simulink model "smc"  (R2015b)
settings: Solver=ode4  StartTime=0.0  StopTime=20  FixedStep=0.0001  RelTol=1e-3
values from neighbouring files (symbols this model uses):
  L = 1    [init.m]
  r = 1    [init.m]
libraries: simulink x1
settings Model: Creator=Subodh  LastModifiedBy=Subodh
settings HardwareCC: ProdWordSize=32  ProdHWDeviceType=Specified

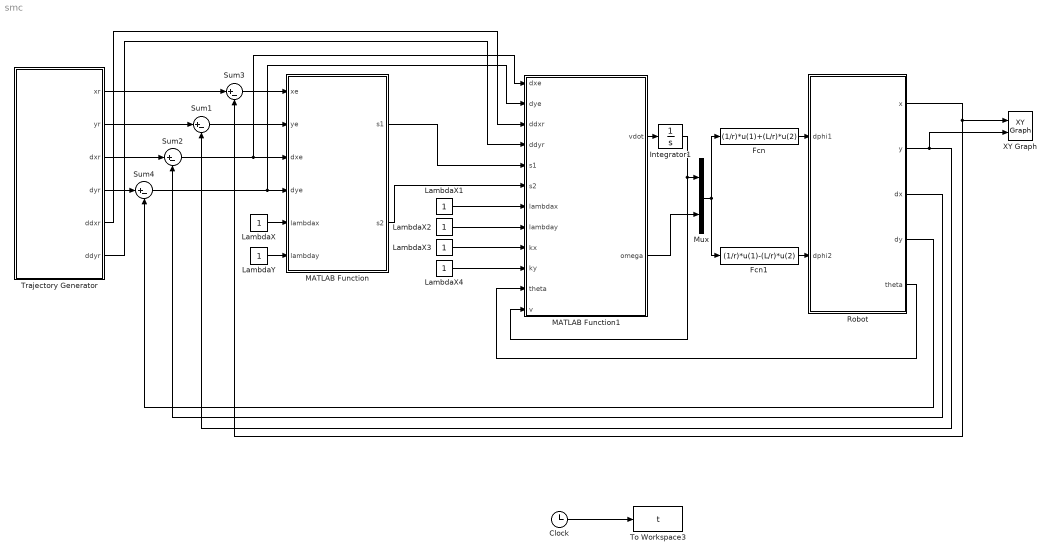
== system smc ==
  "                               LambdaX1" : Constant
  "                               LambdaX2" : Constant
  "                             LambdaX3" : Constant
  "                            LambdaX4" : Constant
  Clock : Clock
  Fcn : Fcn  Expr=(1/r)*u(1)+(L/r)*u(2)
  Fcn1 : Fcn  Expr=(1/r)*u(1)-(L/r)*u(2)
  Integrator1 : Integrator  InitialCondition=1
  LambdaX : Constant
  LambdaY : Constant
  MATLAB Function : MATLAB Function  TreatAsAtomicUnit=on
  MATLAB Function1 : MATLAB Function  TreatAsAtomicUnit=on
  Mux : Mux  Inputs=2
  Robot : Subsystem
  Sum{1..4} (4 alike) : Sum  Inputs=|+-
  To Workspace3 : ToWorkspace  VariableName=t  SampleTime=-1
  Trajectory Generator : Subsystem
  XY Graph : simulink/Sinks/XY Graph  xmin=-2  xmax=2  ymin=-2  ymax=2  st=-1
  wires:
  Clock/1 -> To Workspace3/1
  Trajectory Generator/1(xr) -> Sum3/1
  Robot/1(x) -> XY Graph/1, Sum3/2
  Trajectory Generator/2(yr) -> Sum1/1
  Robot/2(y) -> XY Graph/2, Sum1/2
  Trajectory Generator/3(dxr) -> Sum2/1
  Robot/3(dx) -> Sum2/2
  Trajectory Generator/4(dyr) -> Sum4/1
  Robot/4(dy) -> Sum4/2
  Sum1/1 -> MATLAB Function/2(ye)
  Sum3/1 -> MATLAB Function/1(xe)
  Sum2/1 -> MATLAB Function1/1(dxe), MATLAB Function/3(dxe)
  Sum4/1 -> MATLAB Function1/2(dye), MATLAB Function/4(dye)
  LambdaX/1 -> MATLAB Function/5(lambdax)
  LambdaY/1 -> MATLAB Function/6(lambday)
  MATLAB Function1/1(vdot) -> Integrator1/1
  Integrator1/1 -> Mux/1, MATLAB Function1/12(v)
  Trajectory Generator/5(ddxr) -> MATLAB Function1/3(ddxr)
  Trajectory Generator/6(ddyr) -> MATLAB Function1/4(ddyr)
  Robot/5(theta) -> MATLAB Function1/11(theta)
  "                               LambdaX1"/1 -> MATLAB Function1/7(lambdax)
  "                               LambdaX2"/1 -> MATLAB Function1/8(lambday)
  "                             LambdaX3"/1 -> MATLAB Function1/9(kx)
  "                            LambdaX4"/1 -> MATLAB Function1/10(ky)
  MATLAB Function/1(s1) -> MATLAB Function1/5(s1)
  MATLAB Function/2(s2) -> MATLAB Function1/6(s2)
  Fcn/1 -> Robot/1(dphi1)
  MATLAB Function1/2(omega) -> Mux/2
  Mux/1 -> Fcn/1, Fcn1/1
  Fcn1/1 -> Robot/2(dphi2)

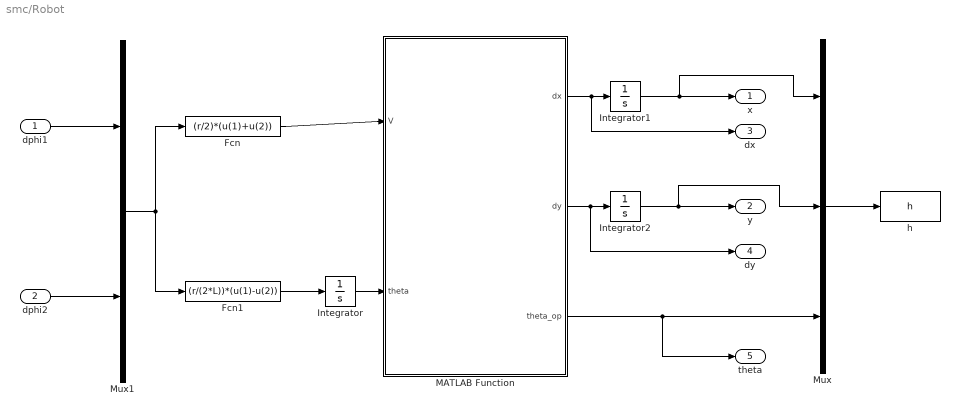
== system smc/Robot ==
  dphi1 : Inport
  dphi2 : Inport  Port=2
  Fcn : Fcn  Expr=(r/2)*(u(1)+u(2))
  Fcn1 : Fcn  Expr=(r/(2*L))*(u(1)-u(2))
  Integrator : Integrator
  Integrator1 : Integrator
  Integrator2 : Integrator
  MATLAB Function : MATLAB Function  TreatAsAtomicUnit=on
  Mux : Mux  Inputs=3
  Mux1 : Mux  Inputs=2
  h : ToWorkspace  VariableName=h  SampleTime=-1
  x : Outport
  y : Outport  Port=2
  dx : Outport  Port=3
  dy : Outport  Port=4
  theta : Outport  Port=5
  wires:
  Integrator1/1 -> Mux/1, x/1
  Integrator/1 -> MATLAB Function/2(theta)
  MATLAB Function/1(dx) -> dx/1, Integrator1/1
  MATLAB Function/2(dy) -> dy/1, Integrator2/1
  Integrator2/1 -> Mux/2, y/1
  MATLAB Function/3(theta_op) -> theta/1, Mux/3
  Mux/1 -> h/1
  dphi2/1 -> Mux1/2
  dphi1/1 -> Mux1/1
  Fcn/1 -> MATLAB Function/1(V)
  Fcn1/1 -> Integrator/1
  Mux1/1 -> Fcn/1, Fcn1/1

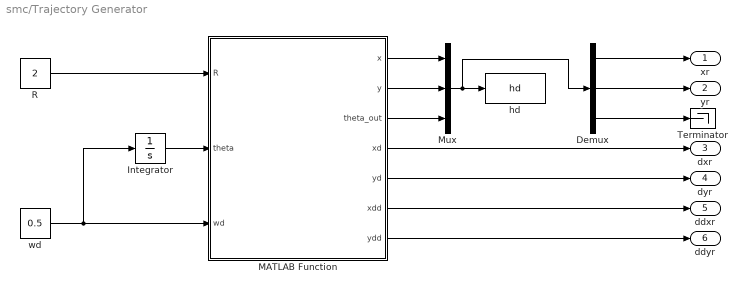
== system smc/Trajectory Generator ==
  Demux : Demux  Outputs=3
  Integrator : Integrator
  MATLAB Function : MATLAB Function  TreatAsAtomicUnit=on
  Mux : Mux  Inputs=3
  R : Constant  Value=2
  Terminator : Terminator
  hd : ToWorkspace  VariableName=hd  SampleTime=-1
  wd : Constant  Value=0.5
  xr : Outport
  yr : Outport  Port=2
  dxr : Outport  Port=3
  dyr : Outport  Port=4
  ddxr : Outport  Port=5
  ddyr : Outport  Port=6
  wires:
  MATLAB Function/4(xd) -> dxr/1
  MATLAB Function/5(yd) -> dyr/1
  MATLAB Function/6(xdd) -> ddxr/1
  MATLAB Function/7(ydd) -> ddyr/1
  R/1 -> MATLAB Function/1(R)
  wd/1 -> Integrator/1, MATLAB Function/3(wd)
  Integrator/1 -> MATLAB Function/2(theta)
  MATLAB Function/1(x) -> Mux/1
  MATLAB Function/2(y) -> Mux/2
  MATLAB Function/3(theta_out) -> Mux/3
  Mux/1 -> Demux/1, hd/1
  Demux/1 -> xr/1
  Demux/2 -> yr/1
  Demux/3 -> Terminator/1

== matlab function smc/Robot/MATLAB Function ==
  data: V input; theta input; dx output; dy output; theta_op output
function [dx,dy,theta_op] = fcn(V,theta)
%#codegen
dx=V*cos(theta);
dy=V*sin(theta);
theta_op=theta;
end

== matlab function smc/Trajectory Generator/MATLAB Function ==
  data: x output; R input; y output; theta_out output; theta input; wd input; xd output; yd output; xdd output; ydd output
function [x,y,theta_out,xd,yd,xdd,ydd] = fcn(R,theta,wd)
%#codegen
x=R*cos(theta);
y=R*sin(theta);
xd=-R*wd*sin(theta);
yd=R*wd*cos(theta);
xdd=-R*(wd^2)*cos(theta);
ydd=-R*(wd^2)*sin(theta);
theta_out=theta+pi/2;
end

== matlab function smc/MATLAB Function ==
  data: xe input; s1 output; ye input; dxe input; dye input; lambdax input; lambday input; s2 output
function [s1,s2] = fcn(xe,ye,dxe,dye,lambdax,lambday)
%#codegen

s1=dxe+lambdax*xe;
s2=dye+lambday*ye;


end

== matlab function smc/MATLAB Function1 ==
  data: dxe input; dye input; ddxr input; ddyr input; s1 input; s2 input; lambdax input; lambday input; kx input; ky input; theta input; v input; vdot output; omega output
function [vdot,omega] = fcn(dxe,dye,ddxr,ddyr,s1,s2,lambdax,lambday,kx,ky,theta,v)
%#codegen


alpha=[ddxr+lambdax*dxe;ddyr+lambday*dye];
beta=[-cos(theta)  v*sin(theta);
      -sin(theta) -v*cos(theta)];
  
u=inv(beta)*([-kx*sign(s1);-ky*sign(s2)]-alpha);

vdot=u(1);
omega=u(2);
end
